simulink model "analysis_sideslip_angre"  (R2019b)
settings: Solver=VariableStepAuto  StartTime=0.0  StopTime=0.3  RelTol=1e-3
values from neighbouring files (symbols this model uses):
  a0 = a11.*a22 - a12.*a21    [coefficien_lateral_accelration.m]    (also in coefficien_sideslip_angre.m; coefficien_turning_trajectory.m; coefficien_yawrate.m)
  a1 = -a11-a22    [coefficien_lateral_accelration.m]    (also in coefficien_sideslip_angre.m; coefficien_turning_trajectory.m; coefficien_yawrate.m)
  b0 = a21.*b11 - a11.*b21    [coefficien_lateral_accelration.m]    (also in coefficien_sideslip_angre.m = a12.*b21 - a22.*b11; coefficien_turning_trajectory.m; coefficien_yawrate.m)
  b1 = a12.*b21 - a22.*b11 + b21    [coefficien_lateral_accelration.m]    (also in coefficien_sideslip_angre.m = b11; coefficien_turning_trajectory.m; coefficien_yawrate.m = b21)
libraries: cstblocks x1
settings Model: Creator=Natsu Nakagawa  LastModifiedBy=Natsu Nakagawa

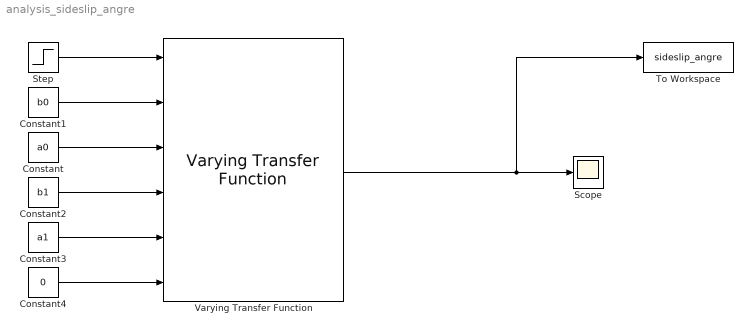
== system analysis_sideslip_angre ==
  Constant : Constant  Value=a0
  Constant1 : Constant  Value=b0
  Constant2 : Constant  Value=b1
  Constant3 : Constant  Value=a1
  Constant4 : Constant  Value=0
  Scope : Scope
  Step : Step  Time=0  SampleTime=0
  To Workspace : ToWorkspace  VariableName=sideslip_angre  SaveFormat=Timeseries  SampleTime=-1
  Varying Transfer Function : cstblocks/Linear Parameter Varying/Varying Transfer Function  N=2
      settings: SourceProductName=Control System Toolbox
  wires:
  Constant4/1 -> Varying Transfer Function/6
  Constant3/1 -> Varying Transfer Function/5
  Constant1/1 -> Varying Transfer Function/2
  Constant2/1 -> Varying Transfer Function/4
  Constant/1 -> Varying Transfer Function/3
  Step/1 -> Varying Transfer Function/1
  Varying Transfer Function/1 -> To Workspace/1, Scope/1
